simulink model "Mo_hinh_DC_motor"  (R2019a)
settings: Solver=VariableStepAuto  StartTime=0.0  StopTime=0.1  RelTol=1e-3
libraries: powerlib x1
settings Model: Creator=Admin  LastModifiedBy=Admin

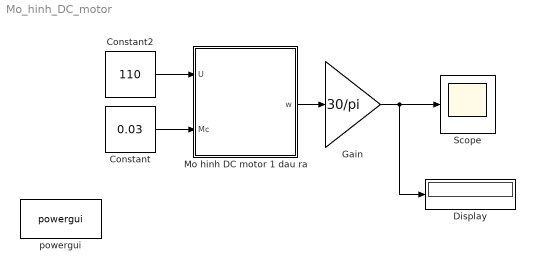
== system Mo_hinh_DC_motor ==
  Constant : Constant  Value=0.03
  Constant2 : Constant  Value=110
  Display : Display
  Gain : Gain  Gain=30/pi
  "Mo hinh DC motor 1 dau ra " : Subsystem  mask{P=1, Ua=110, Uf=110, Ia=9.96, n=3000, Ra=0.561, Rf=500, J=0.8, Cx=30}
      mask prompts: P "Cong suat dinh muc cua dong co"; Ua "Dien ap phan ung dinh muc"; Uf "Dien ap kich tu dinh muc"; Ia "Dong dien phan ung dinh muc"; n "Toc do dinh muc"; Ra "Dien tro cuon day phan ung"; Rf "Dien tro cuon day kich tu"; J "Momen quan tinh"
      mask init:
      | La=(30*Ua*Cx)/(pi*n*Ia)
      | M=(30*P)/(pi*n)
      | If=Uf/Rf
      | Km=M/Ia
      | Ke=30*(Ua-Ra*Ia)/(pi*n)
      | Ta=La/Ra
      mask Display: image('C:\Users\Admin\Pictures\Capture.PNG');
  Scope : Scope
  powergui : powerlib/powergui  Priority=1  SimulationMode=Continuous  SampleTime=50e-6  frequency=60  Iterations=50  frequencyindice=60  Pbase=100e6  ErrMax=1e-4  UnitsV=kV  UnitsW=MW  buscounter=0  FunctionMessages=off  echomessages=off  EnableUseOfTLC=off  CurrentSourceSwitches=off  DisableSnubberDevices=off  DisableRonSwitches=off  DisableVfSwitches=off  DisplayEquations=off  AutomaticDiscreteSolvers=off  SolverType=Tustin/Backward Euler (TBE)  Interpol=off  ExternalGateDelay=off  methode=off  Ts=100  x0status=blocks  SPID=on  SwTol=0  HookPort=off  NonlinearTolerance=0  nMaxIteration=15  ContinueOnMaxIteration=off  RestoreLinks=warning  ResistiveCurrentMeasurement=off  Frange=[0:2:500]  Ylog=off  Xlog=on  ShowGrid=off  save=off  variable=ZData  structure=0  ZoomFFT=off  StartTime=0.0  cycles=1  DisplayStyle=1  fundamental=60  FreqAxis=off  MaxFrequency=1000  frequencyindicesteady=1  RmsSteady=1  display=off
      settings: SourceProductName=Simscape Electrical
  wires:
  Constant/1 -> "Mo hinh DC motor 1 dau ra "/2(Mc)
  Gain/1 -> Display/1, Scope/1
  "Mo hinh DC motor 1 dau ra "/1("w ") -> Gain/1
  Constant2/1 -> "Mo hinh DC motor 1 dau ra "/1(U)

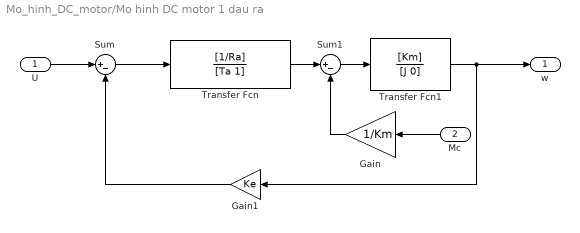
== system Mo_hinh_DC_motor/Mo hinh DC motor 1 dau ra  ==
  U : Inport
  Mc : Inport  Port=2
  Gain : Gain  Gain=1/Km
  Gain1 : Gain  Gain=Ke
  Sum : Sum  Inputs=|+-
  Sum1 : Sum  Inputs=|+-
  Transfer Fcn : TransferFcn  Numerator=[1/Ra]  Denominator=[Ta 1]
  Transfer Fcn1 : TransferFcn  Numerator=[Km]  Denominator=[J 0]
  "w " : Outport
  wires:
  U/1 -> Sum/1
  Transfer Fcn/1 -> Sum1/1
  Sum/1 -> Transfer Fcn/1
  Gain/1 -> Sum1/2
  Mc/1 -> Gain/1
  Transfer Fcn1/1 -> "w "/1, Gain1/1
  Gain1/1 -> Sum/2
  Sum1/1 -> Transfer Fcn1/1
